simulink subsystem "quat2DCM"  (R2024b)
settings: Solver=VariableStepAuto  StartTime=0.0  StopTime=10.0  RelTol=1e-3
settings Model: Creator=ricca  LastModifiedBy=ricca

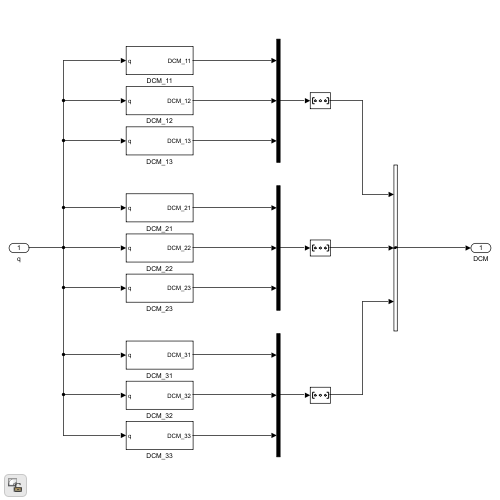
[thumbnail: Simulink's stored preview of the top-level diagram]
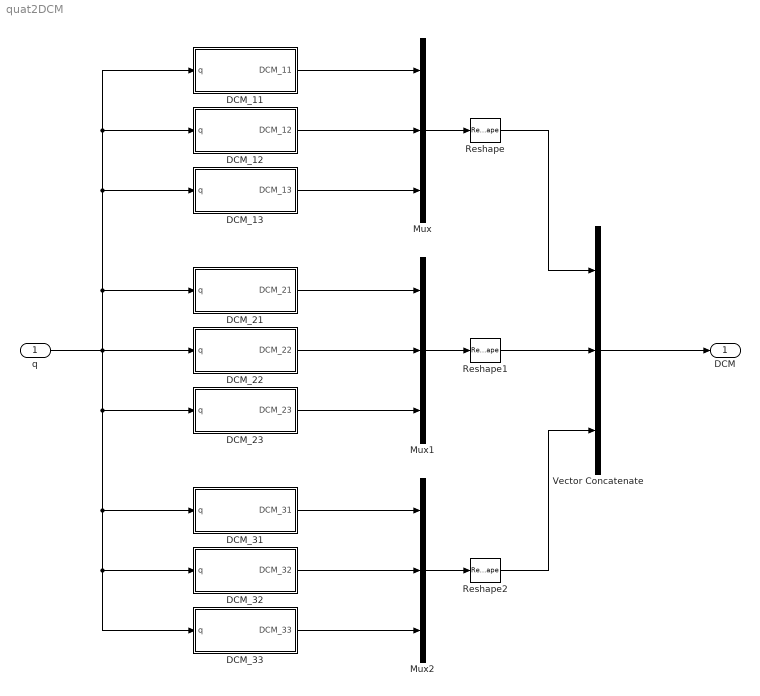
== system quat2DCM ==
  q : Inport
  DCM_11 : Subsystem
  DCM_12 : Subsystem
  DCM_13 : Subsystem
  DCM_21 : Subsystem
  DCM_22 : Subsystem
  DCM_23 : Subsystem
  DCM_31 : Subsystem
  DCM_32 : Subsystem
  DCM_33 : Subsystem
  Mux : Mux  Inputs=3
  Mux1 : Mux  Inputs=3
  Mux2 : Mux  Inputs=3
  Reshape : Reshape  OutputDimensionality=Row vector (2-D)
  Reshape1 : Reshape  OutputDimensionality=Row vector (2-D)
  Reshape2 : Reshape  OutputDimensionality=Row vector (2-D)
  Vector Concatenate : Concatenate  NumInputs=3  Mode=Multidimensional array
  DCM : Outport
  wires:
  q/1 -> DCM_21/1(q), DCM_13/1(q), DCM_12/1(q), DCM_11/1(q), DCM_23/1(q), DCM_31/1(q), DCM_32/1(q), DCM_33/1(q), DCM_22/1(q)
  Mux/1 -> Reshape/1
  Mux1/1 -> Reshape1/1
  Mux2/1 -> Reshape2/1
  Reshape2/1 -> Vector Concatenate/3
  Reshape1/1 -> Vector Concatenate/2
  Reshape/1 -> Vector Concatenate/1
  Vector Concatenate/1 -> DCM/1
  DCM_11/1(DCM_11) -> Mux/1
  DCM_12/1(DCM_12) -> Mux/2
  DCM_13/1(DCM_13) -> Mux/3
  DCM_21/1(DCM_21) -> Mux1/1
  DCM_22/1(DCM_22) -> Mux1/2
  DCM_23/1(DCM_23) -> Mux1/3
  DCM_31/1(DCM_31) -> Mux2/1
  DCM_32/1(DCM_32) -> Mux2/2
  DCM_33/1(DCM_33) -> Mux2/3

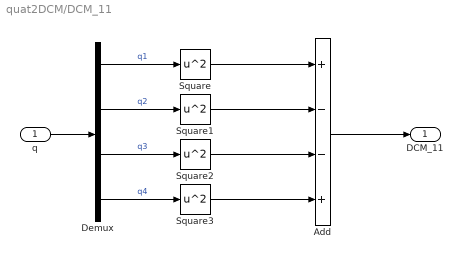
== system quat2DCM/DCM_11 ==
  q : Inport
  Add : Sum  Inputs=+--+
  Demux : Demux
  Square{,1..3} (4 alike) : Math  Operator=square
  DCM_11 : Outport
  wires:
  Square3/1 -> Add/4
  Square2/1 -> Add/3
  Square1/1 -> Add/2
  Square/1 -> Add/1
  Add/1 -> DCM_11/1
  q/1 -> Demux/1
  Demux/2 -> Square1/1  "q2"
  Demux/1 -> Square/1  "q1"
  Demux/3 -> Square2/1  "q3"
  Demux/4 -> Square3/1  "q4"

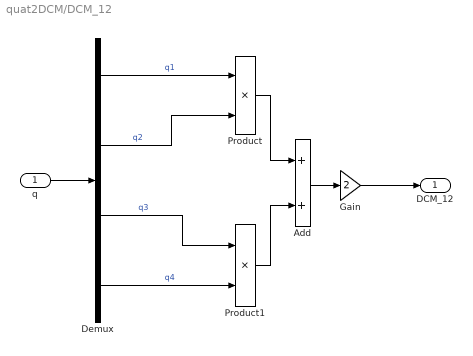
== system quat2DCM/DCM_12 ==
  q : Inport
  Add : Sum
  Demux : Demux
  Gain : Gain  Gain=2
  Product : Product
  Product1 : Product
  DCM_12 : Outport
  wires:
  Product1/1 -> Add/2
  Product/1 -> Add/1
  Gain/1 -> DCM_12/1
  Add/1 -> Gain/1
  q/1 -> Demux/1
  Demux/2 -> Product/2  "q2"
  Demux/1 -> Product/1  "q1"
  Demux/3 -> Product1/1  "q3"
  Demux/4 -> Product1/2  "q4"

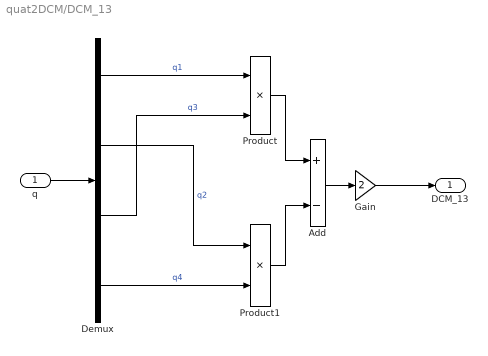
== system quat2DCM/DCM_13 ==
  q : Inport
  Add : Sum  Inputs=+-
  Demux : Demux
  Gain : Gain  Gain=2
  Product : Product
  Product1 : Product
  DCM_13 : Outport
  wires:
  Gain/1 -> DCM_13/1
  Add/1 -> Gain/1
  Product/1 -> Add/1
  Product1/1 -> Add/2
  Demux/2 -> Product1/1  "q2"
  Demux/1 -> Product/1  "q1"
  Demux/4 -> Product1/2  "q4"
  q/1 -> Demux/1
  Demux/3 -> Product/2  "q3"

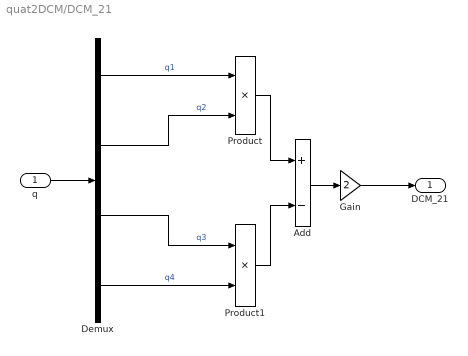
== system quat2DCM/DCM_21 ==
  q : Inport
  Add : Sum  Inputs=+-
  Demux : Demux
  Gain : Gain  Gain=2
  Product : Product
  Product1 : Product
  DCM_21 : Outport
  wires:
  Demux/4 -> Product1/2  "q4"
  Demux/3 -> Product1/1  "q3"
  Demux/2 -> Product/2  "q2"
  Demux/1 -> Product/1  "q1"
  Add/1 -> Gain/1
  q/1 -> Demux/1
  Product/1 -> Add/1
  Gain/1 -> DCM_21/1
  Product1/1 -> Add/2

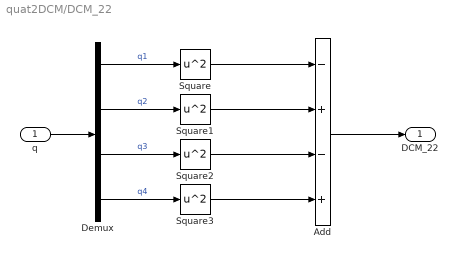
== system quat2DCM/DCM_22 ==
  q : Inport
  Add : Sum  Inputs=-+-+
  Demux : Demux
  Square{,1..3} (4 alike) : Math  Operator=square
  DCM_22 : Outport
  wires:
  q/1 -> Demux/1
  Add/1 -> DCM_22/1
  Demux/2 -> Square1/1  "q2"
  Square/1 -> Add/1
  Demux/1 -> Square/1  "q1"
  Square3/1 -> Add/4
  Demux/3 -> Square2/1  "q3"
  Demux/4 -> Square3/1  "q4"
  Square2/1 -> Add/3
  Square1/1 -> Add/2

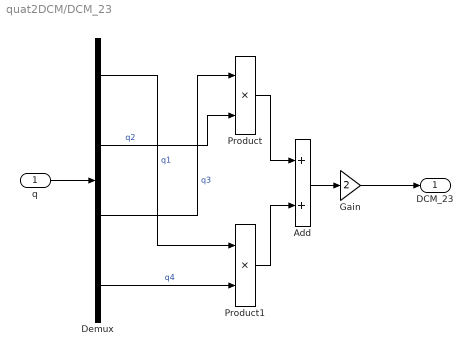
== system quat2DCM/DCM_23 ==
  q : Inport
  Add : Sum
  Demux : Demux
  Gain : Gain  Gain=2
  Product : Product
  Product1 : Product
  DCM_23 : Outport
  wires:
  Demux/4 -> Product1/2  "q4"
  Demux/1 -> Product1/1  "q1"
  Demux/3 -> Product/1  "q3"
  Demux/2 -> Product/2  "q2"
  Add/1 -> Gain/1
  q/1 -> Demux/1
  Product/1 -> Add/1
  Gain/1 -> DCM_23/1
  Product1/1 -> Add/2

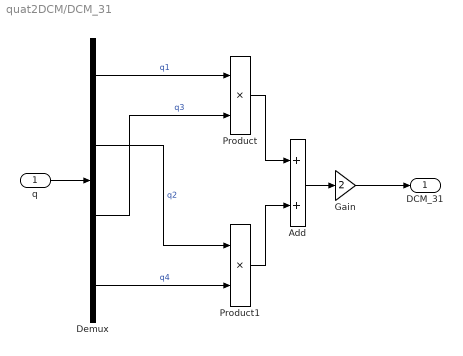
== system quat2DCM/DCM_31 ==
  q : Inport
  Add : Sum
  Demux : Demux
  Gain : Gain  Gain=2
  Product : Product
  Product1 : Product
  DCM_31 : Outport
  wires:
  Demux/3 -> Product/2  "q3"
  Demux/2 -> Product1/1  "q2"
  Demux/1 -> Product/1  "q1"
  Add/1 -> Gain/1
  q/1 -> Demux/1
  Product/1 -> Add/1
  Gain/1 -> DCM_31/1
  Product1/1 -> Add/2
  Demux/4 -> Product1/2  "q4"

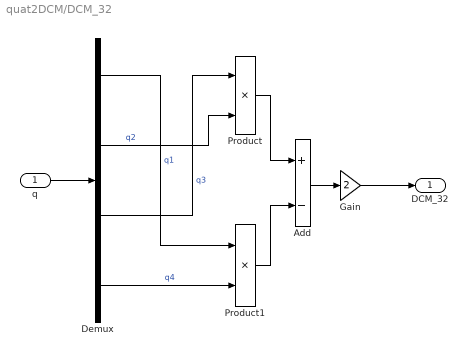
== system quat2DCM/DCM_32 ==
  q : Inport
  Add : Sum  Inputs=+-
  Demux : Demux
  Gain : Gain  Gain=2
  Product : Product
  Product1 : Product
  DCM_32 : Outport
  wires:
  Demux/1 -> Product1/1  "q1"
  Demux/3 -> Product/1  "q3"
  Demux/2 -> Product/2  "q2"
  Add/1 -> Gain/1
  q/1 -> Demux/1
  Product/1 -> Add/1
  Gain/1 -> DCM_32/1
  Product1/1 -> Add/2
  Demux/4 -> Product1/2  "q4"

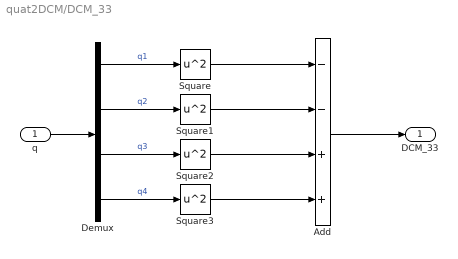
== system quat2DCM/DCM_33 ==
  q : Inport
  Add : Sum  Inputs=--++
  Demux : Demux
  Square{,1..3} (4 alike) : Math  Operator=square
  DCM_33 : Outport
  wires:
  q/1 -> Demux/1
  Add/1 -> DCM_33/1
  Demux/2 -> Square1/1  "q2"
  Square/1 -> Add/1
  Demux/1 -> Square/1  "q1"
  Square3/1 -> Add/4
  Demux/3 -> Square2/1  "q3"
  Demux/4 -> Square3/1  "q4"
  Square2/1 -> Add/3
  Square1/1 -> Add/2
